simulink model "PANCb"  (R2020a)
settings: Solver=ode45  StartTime=0.0  StopTime=10.0  RelTol=1e-3  EnableMultiTasking=on
settings Model: Creator=adeca  LastModifiedBy=Arnaldo
settings DataIOCC: LimitDataPoints=on  SaveFormat=Array  SignalLoggingSaveFormat=ModelDataLogs  ReturnWorkspaceOutputs=off
settings OptimizationCC: ExpressionDepthLimit=2147483647  InitFltsAndDblsToZero=on  LifeSpan=inf
settings DebuggingCC: UnderspecifiedInitializationDetection=Classic  MergeDetectMultiDrivingBlocksExec=none  SolverPrmCheckMsg=warning  FcnCallInpInsideContextMsg=warning  StateNameClashWarn=warning  SFUnexpectedBacktrackingDiag=warning  SFNoUnconditionalDefaultTransitionDiag=warning  SFExecutionAtInitializationDiag=none  ArithmeticOperatorsInVariantConditions=warning
settings HardwareCC: ProdBitPerPointer=32  ProdBitPerSizeT=32  ProdBitPerPtrDiffT=32  ProdLargestAtomicFloat=None  ProdIntDivRoundTo=Undefined  ProdEndianess=Unspecified  ProdWordSize=32  ProdHWDeviceType=32-bit Generic
settings ModelReferenceCC: PropagateSignalLabelsOutOfModel=off
settings SFSimCC: SimUseLocalCustomCode=off  CustomCodeUndefinedFunction=UseInterfaceOnly
settings RTWCC: RTWUseLocalCustomCode=off
settings CodeAppCC: StateflowObjectComments=on
settings GRTTargetCC: TargetLangStandard=C89/C90 (ANSI)  CombineOutputUpdateFcns=off  GRTInterface=on
settings ConfigComp: CovMetricSettings=dw  CovHtmlReporting=on  CovSaveCumulativeToWorkspaceVar=on  CovSaveSingleToWorkspaceVar=on  CovExternalEMLEnable=off

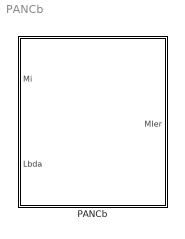
== system PANCb ==
  PANCb : Subsystem  Tag=NAP  Description=Célula de Aprendizagem NAP

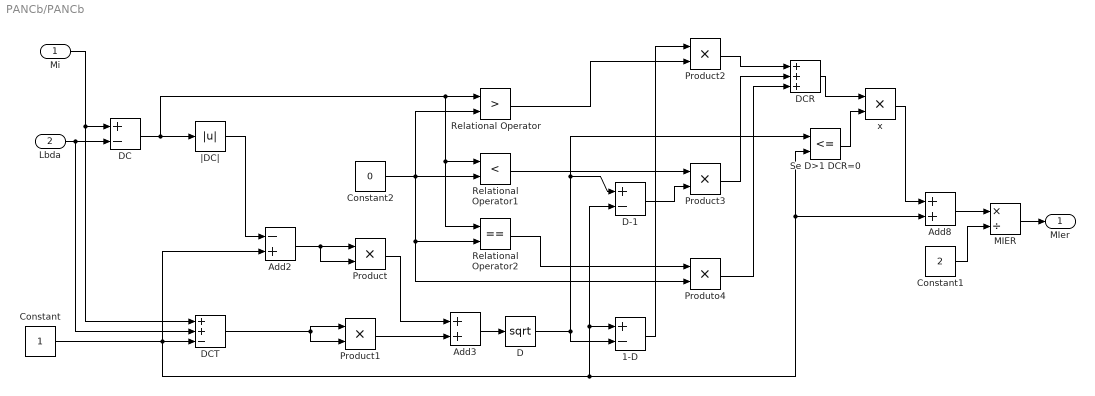
== system PANCb/PANCb ==
  Mi : Inport
  Lbda : Inport  Port=2
  1-D : Sum  Inputs=+-
  Add2 : Sum  Inputs=-+
  Add3 : Sum
  Add8 : Sum
  Constant : Constant
  Constant1 : Constant  Value=2
  Constant2 : Constant  Value=0
  D : Math  Operator=sqrt  SignedPower=on  SaturateOnIntegerOverflow=on
  D-1 : Sum  Inputs=+-
  DC : Sum  Inputs=+-
  DCR : Sum  Inputs=+++
  DCT : Sum  Inputs=++-
  MIER : Product  Inputs=*/
  Product{,1..3} (4 alike) : Product  RndMeth=Zero
  Produto4 : Product  Inputs=**
  Relational Operator : RelationalOperator  Operator=>  OutDataTypeStr=boolean  RndMeth=Nearest
  Relational Operator1 : RelationalOperator  Operator=<  OutDataTypeStr=boolean  RndMeth=Nearest
  Relational Operator2 : RelationalOperator  Operator===  OutDataTypeStr=boolean  RndMeth=Nearest
  Se D>1 DCR=0 : RelationalOperator  Operator=<=  OutDataTypeStr=boolean  RndMeth=Nearest
  x : Product  RndMeth=Zero
  |DC| : Abs
  MIer : Outport  VectorParamsAs1DForOutWhenUnconnected=off
  wires:
  Constant1/1 -> MIER/2
  DC/1 -> Relational Operator/1, Relational Operator1/1, Relational Operator2/1, |DC|/1
  |DC|/1 -> Add2/1
  Add2/1 -> Product/2, Product/1
  DCT/1 -> Product1/1, Product1/2
  Product/1 -> Add3/1
  Product1/1 -> Add3/2
  Relational Operator/1 -> Product2/2
  Constant/1 -> Add2/2, D-1/2, 1-D/1, Add8/2, Se D>1 DCR=0/2, DCT/3
  1-D/1 -> Product2/1
  Product2/1 -> DCR/1
  D-1/1 -> Product3/2
  Relational Operator1/1 -> Product3/1
  Product3/1 -> DCR/2
  Constant2/1 -> Relational Operator/2, Produto4/2, Relational Operator2/2, Relational Operator1/2
  Relational Operator2/1 -> Produto4/1
  Produto4/1 -> DCR/3
  Add8/1 -> MIER/1
  Add3/1 -> D/1
  D/1 -> 1-D/2, D-1/1, Se D>1 DCR=0/1
  Mi/1 -> DC/1, DCT/1
  MIER/1 -> MIer/1
  DCR/1 -> x/1
  Se D>1 DCR=0/1 -> x/2
  x/1 -> Add8/1
  Lbda/1 -> DC/2, DCT/2
